simulink model "punto3d"  (R2018b)
settings: Solver=VariableStepAuto  StartTime=0  StopTime=8  RelTol=1e-3
libraries: dspsrcs4 x3
settings Model: Creator=carta  LastModifiedBy=michha

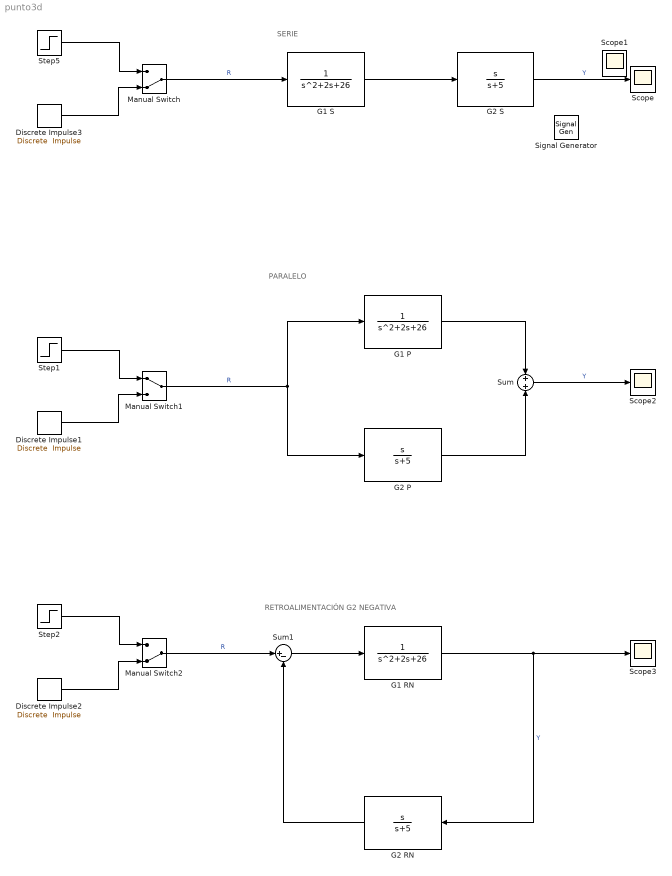
== system punto3d ==
  note: RETROALIMENTACIÓN G2 NEGATIVA
  note: PARALELO
  note: SERIE
  Discrete Impulse1 : dspsrcs4/Discrete  Impulse  Delay=0  SampleTime=0.1  FrameSample=1  OutputFrames=off  dataType=double  isSigned=on  wordLen=16  udDataType=sfix(16)  fracBitsMode=Best precision  numFracBits=15  OutDataTypeStr=double  LastOutDataTypeStr=double
  Discrete Impulse2 : dspsrcs4/Discrete  Impulse  Delay=0  SampleTime=0.1  FrameSample=1  OutputFrames=off  dataType=double  isSigned=on  wordLen=16  udDataType=sfix(16)  fracBitsMode=Best precision  numFracBits=15  OutDataTypeStr=double  LastOutDataTypeStr=double
  Discrete Impulse3 : dspsrcs4/Discrete  Impulse  Delay=0  SampleTime=0.1  FrameSample=1  OutputFrames=off  dataType=double  isSigned=on  wordLen=16  udDataType=sfix(16)  fracBitsMode=Best precision  numFracBits=15  OutDataTypeStr=double  LastOutDataTypeStr=double
  G1 P : TransferFcn  Denominator=[1 2 26]
  G1 RN : TransferFcn  Denominator=[1 2 26]
  G1 S : TransferFcn  Denominator=[1 2 26]
  G2 P : TransferFcn  Numerator=[1 0]  Denominator=[1 5]
  G2 RN : TransferFcn  Numerator=[1 0]  Denominator=[1 5]
  G2 S : TransferFcn  Numerator=[1 0]  Denominator=[1 5]
  Manual Switch : ManualSwitch  CurrentSetting=0
  Manual Switch1 : ManualSwitch
  Manual Switch2 : ManualSwitch  CurrentSetting=0
  Scope{,1..3} (4 alike) : Scope
  Step1 : Step  Time=0  SampleTime=0
  Step2 : Step  Time=0  SampleTime=0
  Step5 : Step  Time=0  SampleTime=0
  Sum : Sum  Inputs=+|+
  Sum1 : Sum  Inputs=|+-
  Signal Generator : SignalGenerator  IOType=siggen
  wires:
  G2 S/1 -> Scope/1  "Y"
  G1 S/1 -> G2 S/1
  Manual Switch/1 -> G1 S/1  "R"
  G1 P/1 -> Sum/1
  G2 P/1 -> Sum/2
  Manual Switch1/1 -> G1 P/1, G2 P/1  "R"
  Sum/1 -> Scope2/1  "Y"
  G1 RN/1 -> G2 RN/1, Scope3/1  "Y"
  G2 RN/1 -> Sum1/2
  Manual Switch2/1 -> Sum1/1  "R"
  Sum1/1 -> G1 RN/1
  Discrete Impulse3/1 -> Manual Switch/2
  Step5/1 -> Manual Switch/1
  Step1/1 -> Manual Switch1/1
  Discrete Impulse1/1 -> Manual Switch1/2
  Step2/1 -> Manual Switch2/1
  Discrete Impulse2/1 -> Manual Switch2/2
